simulink model "Model_1"  (R2020b)
settings: Solver=VariableStepAuto  StartTime=0.0  StopTime=500  RelTol=1e-3
settings Model: Creator=Akarsh  LastModifiedBy=Akarsh

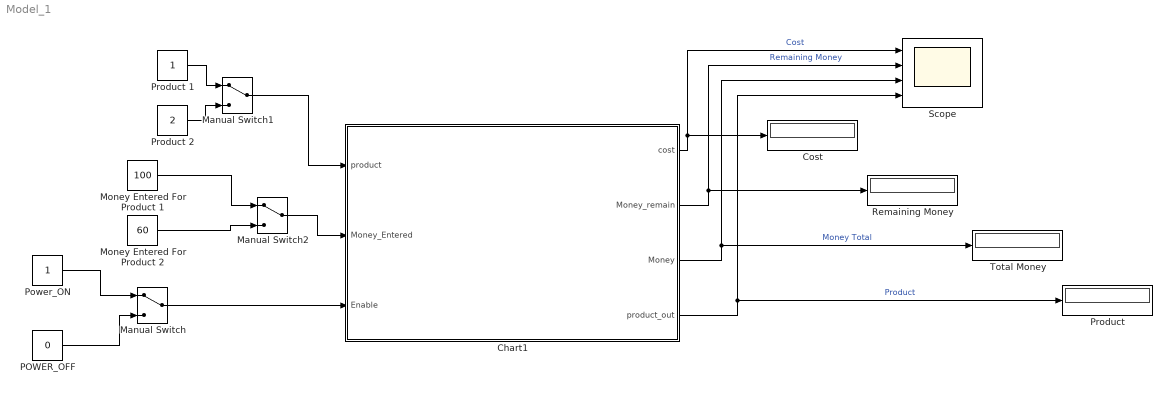
== system Model_1 ==
  Chart1 : Stateflow chart  TreatAsAtomicUnit=on
  Cost : Display
  Manual Switch : ManualSwitch
  Manual Switch1 : ManualSwitch
  Manual Switch2 : ManualSwitch
  Money Entered For Product 1 : Constant  Value=100
  Money Entered For Product 2 : Constant  Value=60
  POWER_OFF : Constant  Value=0
  Power_ON : Constant
  Product : Display
  Product 1 : Constant
  Product 2 : Constant  Value=2
  Remaining Money : Display
  Scope : Scope  NumInputPorts=4
  Total Money : Display
  wires:
  Power_ON/1 -> Manual Switch/1
  POWER_OFF/1 -> Manual Switch/2
  Chart1/2(Money_remain) -> Scope/2, Remaining Money/1  "Remaining Money"
  Chart1/3(Money) -> Scope/3, Total Money/1  "Money Total"
  Chart1/4(product_out) -> Scope/4, Product/1  "Product"
  Chart1/1(cost) -> Scope/1, Cost/1  "Cost"
  Manual Switch/1 -> Chart1/3(Enable)
  Product 1/1 -> Manual Switch1/1
  Product 2/1 -> Manual Switch1/2
  Manual Switch1/1 -> Chart1/1(product)
  Money Entered For Product 1/1 -> Manual Switch2/1
  Money Entered For Product 2/1 -> Manual Switch2/2
  Manual Switch2/1 -> Chart1/2(Money_Entered)

== stateflow chart Model_1/Chart1 ==
  state S0
    Money=0;
    Money_remain=0;
  state Products
  state Product_dispensed
    Money_remain=abs(cost-Money);
  state Money_state
    entry:
    Money=Money+Money_Entered;
    Money_remain=abs(cost-Money);
  (default) -> S0
  S0 -> Products [order 1] : [(product==1) && (Enable)]{cost=100;}
  S0 -> Products [order 2] : [(product==2) && (Enable)]{cost=60}
  Money_state -> Products [order 1] : [(Money<cost)]{product_out=0;}
  Products -> Money_state : [(Money_Entered>0)&&(product_out==0)]
  Product_dispensed -> S0 : [product_out==1]{Money=0;product_out=0;}
  Money_state -> S0 [order 3] : [Enable==0]
  Money_state -> Product_dispensed [order 2] : [Money>=cost]{product_out=1;}
  data: cost output; product input; Money_Entered input; Money_remain output; Money output; product_out output; Enable input
